simulink model "LCK_0112"  (R2018b)
settings: Solver=FixedStepDiscrete  StartTime=0.0  StopTime=inf  FixedStep=0.01  RelTol=1e-3
PostLoadFcn:
  | if any(exist('dsrtsu_mdlpostloadfcn', 'file') ~= 0), dsrtsu_mdlpostloadfcn('Execute', bdroot); end
values from neighbouring files (symbols this model uses):
  C_DEG2RAD = 0.0175    [LCK_Macro.sldd]
  C_KPH2MPS = 0.2778    [LCK_Macro.sldd]
  C_NEARZERO = 0.0001    [LCK_Macro.sldd]
  C_ONE = 1.0    [LCK_Macro.sldd]
  C_RAD2DEG = 57.2958    [LCK_Macro.sldd]
  C_ZERO = 0.0    [LCK_Macro.sldd]
  k_accel_pedal_pos_per_speed_x : value not decoded    [LCK_LogicPara.sldd]
  k_accel_pedal_pos_per_speed_z : value not decoded    [LCK_LogicPara.sldd]
  k_brake_suprress_hold = 1000.0    [LCK_LogicPara.sldd]
  k_driver_appl_torque_filt = 50.0    [LCK_LogicPara.sldd]
  k_driver_suppression_hold_time = 3000.0    [LCK_LogicPara.sldd]
  k_hands_on_wheel_hold_msec = 500.0    [LCK_LogicPara.sldd]
  k_hands_on_wheel_torque_hi = 0.2    [LCK_LogicPara.sldd]
  k_hands_on_wheel_torque_lo = 0.15    [LCK_LogicPara.sldd]
  k_handsoff_delay_cycles = 50.0    [LCK_LogicPara.sldd]
  k_handsoff_torq_Lo_CR = 0.3    [LCK_LogicPara.sldd]
  k_handson_delay_cycles = 5.0    [LCK_LogicPara.sldd]
  k_HighAccel_suppress_hold = 3000.0    [LCK_LogicPara.sldd]
  k_HLR_suprress_hold = 3000.0    [LCK_LogicPara.sldd]
  k_hs_StrAng_CR_threshold_z : value not decoded    [LCK_LogicPara.sldd]
  k_LC_Exit_Switch = 0.0    [LCK_LogicPara.sldd]
  k_LCG_Configured = 1.0    [LCK_LogicPara.sldd]
  k_LCK_A0_Rdy2Act_UseConst = 0.0    [LCK_LogicPara.sldd]
  k_LCK_A0Fac_ActSta : value not decoded    [LCK_CtrlPara.sldd]
  k_LCK_A0Fac_DrvStm : value not decoded    [LCK_CtrlPara.sldd]
  k_LCK_A0Shift_LftCurv : value not decoded    [LCK_CtrlPara.sldd]
  k_LCK_A0Shift_RgtCurv : value not decoded    [LCK_CtrlPara.sldd]
  k_LCK_A0Shift_StraLan = 0.0    [LCK_CtrlPara.sldd]
  k_LCK_A0ShiftFac_Dy_LftCurv : value not decoded    [LCK_CtrlPara.sldd]
  k_LCK_A0ShiftFac_Dy_RgtCurv : value not decoded    [LCK_CtrlPara.sldd]
  k_LCK_A0ShiftFac_Vspd : value not decoded    [LCK_CtrlPara.sldd]
  k_LCK_accel_inhibit_thold = 35.0    [LCK_LogicPara.sldd]
  k_LCK_Active2Ready_Mask = 255.0    [LCK_LogicPara.sldd]
  k_LCK_CvatRateBks : value not decoded    [LCK_CtrlPara.sldd]
  k_LCK_CvatrBks : value not decoded    [LCK_CtrlPara.sldd]
  k_LCK_DFac_Dy : value not decoded    [LCK_CtrlPara.sldd]
  k_LCK_DFac_Dy_Curv : value not decoded    [LCK_CtrlPara.sldd]
  k_LCK_DFac_HaCurCen : value not decoded    [LCK_CtrlPara.sldd]
  k_LCK_DFac_HaCurSid : value not decoded    [LCK_CtrlPara.sldd]
  k_LCK_DFac_HadCurCen : value not decoded    [LCK_CtrlPara.sldd]
  k_LCK_DFac_HadCurSid : value not decoded    [LCK_CtrlPara.sldd]
  k_LCK_DFac_HadStrCen : value not decoded    [LCK_CtrlPara.sldd]
  k_LCK_DFac_HadStrSid : value not decoded    [LCK_CtrlPara.sldd]
  k_LCK_DFac_HaStrCen : value not decoded    [LCK_CtrlPara.sldd]
  k_LCK_DFac_HaStrSid : value not decoded    [LCK_CtrlPara.sldd]
  k_LCK_DFac_Rad : value not decoded    [LCK_CtrlPara.sldd]
  k_LCK_DFac_SA_CurCen : value not decoded    [LCK_CtrlPara.sldd]
  k_LCK_DFac_SA_CurSid : value not decoded    [LCK_CtrlPara.sldd]
  k_LCK_DFac_SA_StrCen : value not decoded    [LCK_CtrlPara.sldd]
  k_LCK_DFac_SA_StrSid : value not decoded    [LCK_CtrlPara.sldd]
  k_LCK_DFac_SS_CurCen : value not decoded    [LCK_CtrlPara.sldd]
  k_LCK_DFac_SS_CurSid : value not decoded    [LCK_CtrlPara.sldd]
  k_LCK_DFac_SS_StrCen : value not decoded    [LCK_CtrlPara.sldd]
  k_LCK_DFac_SS_StrSid : value not decoded    [LCK_CtrlPara.sldd]
  k_LCK_DFac_Vspd : value not decoded    [LCK_CtrlPara.sldd]
  k_LCK_DlyTm_DrvStim = 0.2    [LCK_CtrlPara.sldd]
  k_LCK_DTermMax = 2.0    [LCK_CtrlPara.sldd]
  k_LCK_DyBks_Curv : value not decoded    [LCK_CtrlPara.sldd]
  k_LCK_Enable_POOnly = 1.0    [LCK_LogicPara.sldd]
  k_LCK_Entry_DistBuffer = 0.1    [LCK_LogicPara.sldd]
  k_LCK_Fac_Vspd2RngThr_FalRec = 0.23    [LCK_CtrlPara.sldd]
  k_LCK_Ffw_CvatSwh = 0.0    [LCK_CtrlPara.sldd]
  k_LCK_Ffw_DyBks : value not decoded    [LCK_CtrlPara.sldd]
  k_LCK_Ffw_TimCon_CmdFlt = 0.0    [LCK_CtrlPara.sldd]
  k_LCK_FfwDeltaFac_Rad_Lft : value not decoded    [LCK_CtrlPara.sldd]
  k_LCK_FfwDeltaFac_Rad_Rgt : value not decoded    [LCK_CtrlPara.sldd]
  k_LCK_FfwDeltaFac_Vspd : value not decoded    [LCK_CtrlPara.sldd]
  k_LCK_FfwFac_CvatRate_Lft : value not decoded    [LCK_CtrlPara.sldd]
  k_LCK_FfwFac_CvatRate_Rgt : value not decoded    [LCK_CtrlPara.sldd]
  k_LCK_FfwFac_Dy : value not decoded    [LCK_CtrlPara.sldd]
  k_LCK_FfwFac_Rad_Lft : value not decoded    [LCK_CtrlPara.sldd]
  k_LCK_FfwFac_Rad_Rgt : value not decoded    [LCK_CtrlPara.sldd]
  k_LCK_FfwFac_Vspd : value not decoded    [LCK_CtrlPara.sldd]
  k_LCK_FfwTorq_Cvat : value not decoded    [LCK_CtrlPara.sldd]
  k_LCK_HAFac_ActSta : value not decoded    [LCK_CtrlPara.sldd]
  k_LCK_HAFac_DrvStm : value not decoded    [LCK_CtrlPara.sldd]
  k_LCK_HaloTime = 2000.0    [LCK_LogicPara.sldd]
  k_LCK_HaloTime_Switch = 0.0    [LCK_LogicPara.sldd]
  k_LCK_HARFac_ActSta : value not decoded    [LCK_CtrlPara.sldd]
  k_LCK_HARFac_DrvStm : value not decoded    [LCK_CtrlPara.sldd]
  k_LCK_Hed_DyBks : value not decoded    [LCK_CtrlPara.sldd]
  k_LCK_HedAngDiffX : value not decoded    [LCK_CtrlPara.sldd]
  k_LCK_HedAngRateDiffX : value not decoded    [LCK_CtrlPara.sldd]
  k_LCK_HndsOnWhel_DlyTm_Idl2Rdy = 0.0    [LCK_LogicPara.sldd]
  k_LCK_host_veh_width = 1.86    [LCK_LogicPara.sldd]
  k_LCK_Idle2Ready_Mask = 239.0    [LCK_LogicPara.sldd]
  k_LCK_Junc_SusTime = 1.0    [LCK_LogicPara.sldd]
  k_LCK_KpKdDecSlopeLmt = 10.0    [LCK_CtrlPara.sldd]
  k_LCK_KpKdIncSlopeLmt = 5.0    [LCK_CtrlPara.sldd]
  k_LCK_Lat_Ctrl_DFac_Lft = 1.0    [LCK_CtrlPara.sldd]
  k_LCK_Lat_Ctrl_DFac_Rgt = 1.05    [LCK_CtrlPara.sldd]
  k_LCK_Lat_Ctrl_Kd = 0.8    [LCK_CtrlPara.sldd]
  k_LCK_Lat_Ctrl_Ki = 0.5    [LCK_CtrlPara.sldd]
  k_LCK_Lat_Ctrl_Kp = 0.7    [LCK_CtrlPara.sldd]
  k_LCK_Lat_Ctrl_Kp_NearGain = 0.7    [LCK_CtrlPara.sldd]
  k_LCK_Lat_Ctrl_PFac_Lft = 1.0    [LCK_CtrlPara.sldd]
  k_LCK_Lat_Ctrl_PFac_Rgt = 1.05    [LCK_CtrlPara.sldd]
  k_LCK_Lat_Ctrl_TimCon_CmdFlt = 5.0    [LCK_CtrlPara.sldd]
  k_LCK_Lat_DFac_Rad : value not decoded    [LCK_CtrlPara.sldd]
  k_LCK_Lat_DFac_SS_Cur : value not decoded    [LCK_CtrlPara.sldd]
  k_LCK_Lat_DFac_SS_Str : value not decoded    [LCK_CtrlPara.sldd]
  k_LCK_Lat_DFac_Vspd : value not decoded    [LCK_CtrlPara.sldd]
  k_LCK_Lat_DyBks : value not decoded    [LCK_CtrlPara.sldd]
  k_LCK_Lat_IFac_Rad : value not decoded    [LCK_CtrlPara.sldd]
  k_LCK_Lat_IFac_Vspd : value not decoded    [LCK_CtrlPara.sldd]
  k_LCK_Lat_ILmtFac_Dy_CurvLan : value not decoded    [LCK_CtrlPara.sldd]
  k_LCK_Lat_ILmtFac_Dy_StraLan : value not decoded    [LCK_CtrlPara.sldd]
  k_LCK_Lat_ILmtFac_Rad : value not decoded    [LCK_CtrlPara.sldd]
  k_LCK_Lat_ILmtFac_Rad_NearGain = 1.0    [LCK_CtrlPara.sldd]
  k_LCK_Lat_ILmtFac_Vspd_CurvLan : value not decoded    [LCK_CtrlPara.sldd]
  k_LCK_Lat_ILmtFac_Vspd_StraLan : value not decoded    [LCK_CtrlPara.sldd]
  k_LCK_Lat_ITermLmt_Dy = 1.0    [LCK_CtrlPara.sldd]
  k_LCK_Lat_KpKdDecSlopeLmt = 10.0    [LCK_CtrlPara.sldd]
  k_LCK_Lat_KpKdIncSlopeLmt = 10.0    [LCK_CtrlPara.sldd]
  k_LCK_Lat_PFac_Dy_InnLftCur : value not decoded    [LCK_CtrlPara.sldd]
  k_LCK_Lat_PFac_Dy_InnRgtCur : value not decoded    [LCK_CtrlPara.sldd]
  k_LCK_Lat_PFac_Dy_OutLftCur : value not decoded    [LCK_CtrlPara.sldd]
  k_LCK_Lat_PFac_Dy_OutRgtCur : value not decoded    [LCK_CtrlPara.sldd]
  k_LCK_Lat_PFac_Dy_Str : value not decoded    [LCK_CtrlPara.sldd]
  k_LCK_Lat_PFac_Rad : value not decoded    [LCK_CtrlPara.sldd]
  ... (+153 more)
undefined symbols (not defined in the file or in its folder): k_LCK_CurvBks, K_LCK_SPA0A1A2_LMRngCmp_y
libraries: LateralControl_fcns_lib x58, simulink x24
(part 24 of 45)

== system LCK_0112/Lateral_Control_Module/LCK_State_Ctrl/Det_Driver_Operation/Det_Hands_on_Wheel ==
  note: 50
  TorsionBarTorque : Inport  Description=_GWMH9P3.Latctrl.000_23_
  Abs : Abs  Description=_GWMH9P3.Latctrl.000_31_
  Abs2 : Abs  Description=_GWMH9P3.Latctrl.000_47_
  Constant : Constant  Description=_GWMH9P3.Latctrl.000_49_  Value=k_hands_on_wheel_torque_hi
  Constant3 : Constant  Description=_GWMH9P3.Latctrl.000_50_  Value=k_hands_on_wheel_torque_lo
  Constant4 : Constant  Description=_GWMH9P3.Latctrl.000_51_  Value=C_ONE
  Constant5 : Constant  Description=_GWMH9P3.Latctrl.000_52_  Value=C_ZERO
  Delay_Trig_Cnt : LateralControl_fcns_lib/Delay_Trig_Cnt  Description=_GWMAB30P4.LKAFN.000_28_  SystemSampleTime=-1
  Delay_Trig_Cnt1 : LateralControl_fcns_lib/Delay_Trig_Cnt  Description=_GWMAB30P4.LKAFN.000_28_  SystemSampleTime=-1
  First_Order_Lag_Filter_LIB : LateralControl_fcns_lib/First_Order_Lag_Filter_LIB  SystemSampleTime=-1
  Gain : Gain  Description=_GWMH9P3.Latctrl.000_75_
  Logical Operator8 : Logic  Description=_GWMH9P3.Latctrl.000_54_  AllPortsSameDT=off  OutDataTypeStr=boolean
  ML_TIME_MSEC : Constant  Description=_GWMH9P3.Latctrl.000_83_  Value=ML_TIME_MSEC
  Relational Operator11 : RelationalOperator  Description=_GWMH9P3.Latctrl.000_56_  Operator=<=  OutDataTypeStr=boolean  RndMeth=Nearest
  Relational Operator12 : RelationalOperator  Description=_GWMH9P3.Latctrl.000_57_  Operator=<=  OutDataTypeStr=boolean  RndMeth=Nearest
  Relational Operator13 : RelationalOperator  Description=_GWMH9P3.Latctrl.000_58_  OutDataTypeStr=boolean  RndMeth=Nearest
  Signal_Sustain_With_Clear : LateralControl_fcns_lib/Signal_Sustain_With_Clear  Description=_GWMAB30P4.Latctrl.000_162_  SystemSampleTime=-1
  Subtract : Sum  Description=_GWMH9P3.Latctrl.000_59_  Inputs=+-
  Switch13 : Switch  Description=_GWMH9P3.Latctrl.000_60_  Criteria=u2 ~= 0
  Switch14 : Switch  Description=_GWMH9P3.Latctrl.000_61_  Criteria=u2 ~= 0
  Unit Delay1 : UnitDelay  Description=_GWMH9P3.Latctrl.000_64_  SampleTime=-1
  Unit Delay2 : UnitDelay  Description=_GWMH9P3.Latctrl.000_65_  SampleTime=-1
  k_driver_appl_torque_filt : Constant  Description=_GWMH9P3.Latctrl.000_102_  Value=k_driver_appl_torque_filt
  k_hands_on_wheel_hold_msec : Constant  Description=_GWMH9P3.Latctrl.000_66_  Value=k_hands_on_wheel_hold_msec
  k_handsoff_delay_cycles : Constant  Description=_GWMH9P3.Latctrl.000_67_  Value=k_handsoff_delay_cycles
  k_handsoff_torq_Lo_CR : Constant  Description=_GWMH9P3.Latctrl.000_69_  Value=k_handsoff_torq_Lo_CR
  k_handson_delay_cycles : Constant  Description=_GWMH9P3.Latctrl.000_70_  Value=k_handson_delay_cycles
  zero_exit_cond : Constant  Description=_GWMH9P3.Latctrl.000_71_  Value=C_ZERO
  f_hands_on_wheel : Outport  Description=_GWMAB30P4.Latctrl.000_740_
  wires:
  Delay_Trig_Cnt/1 -> Switch13/2
  Constant/1 -> Relational Operator13/2
  Logical Operator8/1 -> Delay_Trig_Cnt1/1
  TorsionBarTorque/1 -> First_Order_Lag_Filter_LIB/1
  Abs/1 -> Unit Delay2/1, Subtract/1, Relational Operator11/1, Relational Operator13/1
  Signal_Sustain_With_Clear/1 -> Gain/1  "Delphi_Handson"
  Relational Operator13/1 -> Delay_Trig_Cnt/1
  Constant5/1 -> Switch14/1
  ML_TIME_MSEC/1 -> First_Order_Lag_Filter_LIB/3
  Unit Delay2/1 -> Subtract/2
  Abs2/1 -> Relational Operator12/1
  Gain/1 -> f_hands_on_wheel/1  "f_hands_on_wheel"
  Delay_Trig_Cnt1/1 -> Switch14/2
  First_Order_Lag_Filter_LIB/1 -> Abs/1
  Constant4/1 -> Switch13/1
  Constant3/1 -> Relational Operator11/2
  Switch13/1 -> Signal_Sustain_With_Clear/1, Unit Delay1/1
  Subtract/1 -> Abs2/1
  Switch14/1 -> Switch13/3
  k_driver_appl_torque_filt/1 -> First_Order_Lag_Filter_LIB/2
  zero_exit_cond/1 -> Signal_Sustain_With_Clear/3
  Unit Delay1/1 -> Switch14/3
  k_hands_on_wheel_hold_msec/1 -> Signal_Sustain_With_Clear/2
  Relational Operator11/1 -> Logical Operator8/1
  k_handsoff_torq_Lo_CR/1 -> Relational Operator12/2
  k_handsoff_delay_cycles/1 -> Delay_Trig_Cnt1/2
  Relational Operator12/1 -> Logical Operator8/2
  k_handson_delay_cycles/1 -> Delay_Trig_Cnt/2

== system LCK_0112/Lateral_Control_Module/LCK_State_Ctrl/Det_Driver_Operation/Filter_Accel_Pedal ==
  note: LSS_SnvtySet
  note: Detect that accelerator pedal has been pressed greater than X threshold, within the past Y time
  note: The FCM shall inhibit LKA Intevention when the driver is pressing the accelerator pedal (CAN BUS signal Accelerator Actual Position) at a rate greater than Accelerator_Pedal_Rate (default 50.96%/sec) calibration for a calibratible time, then LKA shall be inhibited and stop intervention.
      | The accelerator pedal position value shall be filtered to provide accelerator pedal position rate of change and reject high frequency noise.  There shall be an accelerator_pedal_position_filter_constant calibration available to adjust the filter response characteristic.
  Accel_Pedal_Posn : Inport  Description=_GWMAB30P4.Latctrl.000_102_
  GearLeverPos : Inport  Description=_GWMAB30P4.Latctrl.000_104_  Port=2
  IP_vehicle_speed : Inport  Description=_GWMAB30P4.Latctrl.000_103_  Port=3
  Add2 : Sum  Description=_GWMAB30P3.Latctrl.000_108_  Inputs=+-
  Constant11 : Constant  Description=_GWMAB30P3.Latctrl.000_109_  Value=4
  LSS_SnvtySet : Constant  Description=_GWMAB30P3.Latctrl.000_138_  Value=0
  Logical Operator2 : Logic  Description=_GACA26P3.Latctrl.000_35_  AllPortsSameDT=off  OutDataTypeStr=boolean
  Relational Operator1 : RelationalOperator  Description=_GWMAB30P3.Latctrl.000_119_  Operator===  OutDataTypeStr=boolean  RndMeth=Nearest
  Relational Operator3 : RelationalOperator  Description=_GACA26P3.Latctrl.000_36_  Operator=>  OutDataTypeStr=boolean  RndMeth=Nearest
  accel_pedal_pos_per_speed : Lookup_n-D  Description=_GWMAB30P3.Latctrl.000_124_  NumberOfTableDimensions=1  BreakpointsForDimension1=k_accel_pedal_pos_per_speed_x  IndexSearchMethod=Linear search  Table=k_accel_pedal_pos_per_speed_z  ExtrapMethod=Clip  InputSameDT=on
  k_LCK_accel_inhibit_thold : Constant  Description=_GACA26P3.Latctrl.000_37_  Value=k_LCK_accel_inhibit_thold
  f_LCK_accel_pedal_inhibit : Outport  Description=_GACA26P3.Latctrl.000_38_
  wires:
  Logical Operator2/1 -> f_LCK_accel_pedal_inhibit/1
  Add2/1 -> Relational Operator3/1
  k_LCK_accel_inhibit_thold/1 -> Relational Operator3/2
  Relational Operator3/1 -> Logical Operator2/2
  LSS_SnvtySet/1 -> [LSS_SnvtySet]
  Accel_Pedal_Posn/1 -> [AccPedalPosition]
  IP_vehicle_speed/1 -> [IP_veh_spd_kph]
  [IP_veh_spd_kph] -> accel_pedal_pos_per_speed/1
  [AccPedalPosition] -> Add2/1
  accel_pedal_pos_per_speed/1 -> Add2/2
  GearLeverPos/1 -> [Gear_Pos]
  [Gear_Pos] -> Relational Operator1/1
  Constant11/1 -> Relational Operator1/2
  Relational Operator1/1 -> Logical Operator2/1
